simulink model "pendulum_with_input"  (Simulink 10.1)
settings: Solver=FixedStepAuto  StartTime=0.0  StopTime=stopTime  FixedStep=T  RelTol=1e-3
values from neighbouring files (symbols this model uses):
  b = 50    [init_araba_hiz_kontrol.m]    (also in init_araba_hiz_on_off_kontrol.m; init_araba_hiz_pid_kontrol.m; init_araba_pozisyon_bang_bang_kontrol.m = 250; init_araba_pozisyon_kontrol.m)
  g = 9.8    [init_pendulum.m]    (also in init_pendulum_with_input.m)
  Kd = 195    [init_araba_hiz_kontrol.m]    (also in init_araba_hiz_pid_kontrol.m; init_araba_pozisyon_kontrol.m = 375; init_araba_pozisyon_pid_kontrol.m = 375; init_pendulum_with_input.m = 15)
  Ki = 70    [init_araba_hiz_kontrol.m]    (also in init_araba_hiz_pid_kontrol.m; init_araba_pozisyon_kontrol.m = 0; init_araba_pozisyon_pid_kontrol.m = 0; init_pendulum_with_input.m = 10)
  Kp = 5000    [init_araba_hiz_kontrol.m]    (also in init_araba_hiz_pid_kontrol.m; init_araba_pozisyon_kontrol.m = 20; init_araba_pozisyon_pid_kontrol.m = 20; init_pendulum_with_input.m = 80)
  l = 1    [init_pendulum.m]    (also in init_pendulum_with_input.m)
  m = 1000    [init_araba_hiz_kontrol.m]    (also in init_araba_hiz_on_off_kontrol.m; init_araba_hiz_pid_kontrol.m; init_araba_pozisyon_bang_bang_kontrol.m; init_araba_pozisyon_kontrol.m)
  r = 5    [init_RC_devresi_bang_bang_kontrol.m]    (also in init_araba_hiz_kontrol.m = 90; init_araba_hiz_on_off_kontrol.m = 90; init_araba_hiz_pid_kontrol.m = 90; init_araba_pozisyon_bang_bang_kontrol.m = 1000)
  umax = 100    [init_pendulum_with_input.m]
  umin = -100    [init_pendulum_with_input.m]
  x10 = 0    [init_araba_hiz_kontrol.m]    (also in init_araba_hiz_on_off_kontrol.m; init_araba_hiz_pid_kontrol.m; init_araba_pozisyon_bang_bang_kontrol.m; init_araba_pozisyon_kontrol.m)
  x20 = 0    [init_araba_hiz_kontrol.m]    (also in init_araba_hiz_on_off_kontrol.m; init_araba_hiz_pid_kontrol.m; init_araba_pozisyon_bang_bang_kontrol.m; init_araba_pozisyon_kontrol.m)
libraries: simulink x1
settings Model: Creator=TULPAR  LastModifiedBy=TULPAR
settings DataIOCC: SaveFormat=Dataset  ReturnWorkspaceOutputs=on
settings OptimizationCC: LifeSpan=auto
settings DebuggingCC: UnderspecifiedInitializationDetection=Simplified  MergeDetectMultiDrivingBlocksExec=error  SFUnexpectedBacktrackingDiag=error  SFNoUnconditionalDefaultTransitionDiag=error  SFExecutionAtInitializationDiag=warning  ArithmeticOperatorsInVariantConditions=error
settings HardwareCC: ProdBitPerPointer=64  ProdBitPerSizeT=64  ProdBitPerPtrDiffT=64  ProdLargestAtomicFloat=Float  ProdIntDivRoundTo=Zero  ProdEndianess=LittleEndian  ProdWordSize=64  ProdHWDeviceType=Intel->x86-64 (Windows64)
settings ModelReferenceCC: PropagateSignalLabelsOutOfModel=on
settings SFSimCC: SimUseLocalCustomCode=on  CustomCodeUndefinedFunction=FilterOut
settings RTWCC: RTWUseLocalCustomCode=on
settings CodeAppCC: StateflowObjectComments=off
settings GRTTargetCC: TargetLangStandard=C99 (ISO)  CombineOutputUpdateFcns=on  GRTInterface=off
settings ConfigComp: CovMetricSettings=dwe  CovHtmlReporting=off  CovSaveCumulativeToWorkspaceVar=off  CovSaveSingleToWorkspaceVar=off  CovExternalEMLEnable=on

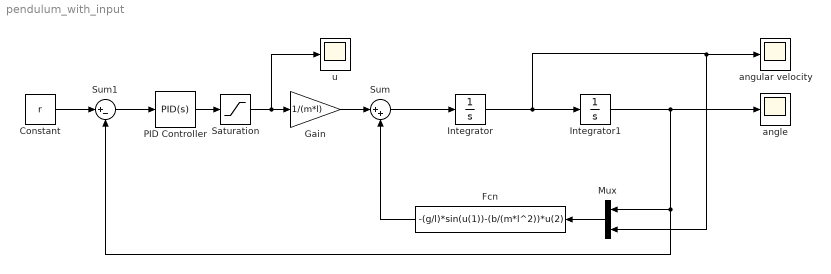
== system pendulum_with_input ==
  Constant : Constant  Value=r
  Fcn : Fcn  Expr=-(g/l)*sin(u(1))-(b/(m*l^2))*u(2)
  Gain : Gain  Gain=1/(m*l)
  Integrator : Integrator  InitialCondition=x20
  Integrator1 : Integrator  InitialCondition=x10
  Mux : Mux  Inputs=2
  PID Controller : simulink/Continuous/PID Controller  Controller=PID  Form=Parallel  TimeDomain=Continuous-time  UseExternalTs=off  SampleTime=-1  IntegratorMethod=Forward Euler  FilterMethod=Forward Euler  ControllerParametersSource=internal  P=Kp  I=Ki  D=Kd  UseFilter=on  N=100  TunerSelectOption=Transfer Function Based (PID Tuner App)  InitialConditionSource=internal  InitialConditionForIntegrator=0  InitialConditionForFilter=0  DifferentiatorICPrevScaledInput=0  ExternalReset=none  TrackingMode=off  Kt=1  LimitOutput=off  UpperSaturationLimit=inf  LowerSaturationLimit=-inf  LinearizeAsGain=on  AntiWindupMode=none  Kb=1  POutMin=[]  POutMax=[]  IOutMin=[]  IOutMax=[]  DOutMin=[]  DOutMax=[]  NOutMin=[]  NOutMax=[]  SumOutMin=[]  SumOutMax=[]  SaturationOutMin=[]  SaturationOutMax=[]  PParamMin=[]  PParamMax=[]  IParamMin=[]  IParamMax=[]  DParamMin=[]  DParamMax=[]  NParamMin=[]  NParamMax=[]  KbParamMin=[]  KbParamMax=[]  KtParamMin=[]  KtParamMax=[]  KbOutMin=[]  KbOutMax=[]  KtOutMin=[]  KtOutMax=[]  IntegratorOutMin=[]  IntegratorOutMax=[]  FilterOutMin=[]  FilterOutMax=[]  SumI1OutMin=[]  SumI1OutMax=[]  SumI2OutMin=[]  SumI2OutMax=[]  SumI3OutMin=[]  SumI3OutMax=[]  SumI4OutMin=[]  SumI4OutMax=[]  SumDOutMin=[]  SumDOutMax=[]  DifferentiatorOutMin=[]  DifferentiatorOutMax=[]  FilterDiffOutCoefMin=[]  FilterDiffOutCoefMax=[]  ReciprocalOutMin=[]  ReciprocalOutMax=[]  SumDenOutMin=[]  SumDenOutMax=[]  SumNumOutMin=[]  SumNumOutMax=[]  DivideOutMin=[]  DivideOutMax=[]  UdiffTsProdOutMin=[]  UdiffTsProdOutMax=[]  NTsProdOutMin=[]  NTsProdOutMax=[]  UintegralTsProdOutMin=[]  UintegralTsProdOutMax=[]  UngainTsProdOutMin=[]  UngainTsProdOutMax=[]  IntegratorContinuousStateAttributes=''  IntegratorStateMustResolveToSignalObject=off  IntegratorRTWStateStorageClass=Auto  FilterContinuousStateAttributes=''  FilterStateMustResolveToSignalObject=off  FilterRTWStateStorageClass=Auto  ParallelPVariant=InternalParameters  IdealPVariant=Disabled  IVariant=InternalParameters  DVariant=InternalParameters  IntegratorVariant=Continuous  SatVariant=Disabled  AWVariant=Passthrough  PCopyVariant=Disabled  TRVariant=Disabled  FdbkBlocksVariant=Forward  IdealPFdbkVariant=Disabled  SatFdbkVariant=Disabled  DerivativeFilterVariant=ContFilter  NVariant=InternalParameters  NCopyVariant=Disabled  FilterICVariant=InternalICsFilter  IntegratorICVariant=InternalICs  ExternalResetVariant=Disabled  TRSumVariant=Passthrough  SumFdbkVariant=Disabled  SumVariant=Sum_PID  TsampFilterVariant=InternalTs  TsampNgainVariant=Passthrough  TsampIntegralVariant=Passthrough
  Saturation : Saturate  UpperLimit=umax  LowerLimit=umin
  Sum : Sum  Inputs=|++
  Sum1 : Sum  Inputs=|+-
  angle : Scope
  angular velocity : Scope
  u : Scope
  wires:
  Integrator1/1 -> angle/1, Sum1/2, Mux/1
  Mux/1 -> Fcn/1
  Integrator/1 -> Integrator1/1, angular velocity/1, Mux/2
  Fcn/1 -> Sum/2
  Gain/1 -> Sum/1
  Constant/1 -> Sum1/1
  Sum1/1 -> PID Controller/1
  Sum/1 -> Integrator/1
  PID Controller/1 -> Saturation/1
  Saturation/1 -> u/1, Gain/1
